simulink model "Stereotypes_Example"  (R2024a)
settings: Solver=VariableStepAuto  StartTime=0.0  StopTime=10.0  RelTol=1e-3
model workspace (MAT data in the model file):
  Var = 0
  architecture_gsCommands : Simulink.Bus (value not decoded)
  ctrlSrfcDeflection : Simulink.Bus (value not decoded)
  gs_commands_bus : Simulink.Bus (value not decoded)
  lightCmds : Simulink.Bus (value not decoded)
  mission_item_bus : Simulink.Bus (value not decoded)
  operatorCmds : Simulink.Bus (value not decoded)
  param_value_bus : Simulink.Bus (value not decoded)
(part 2 of 2)

== system Stereotypes_Example/Propulsion/Engine/ECU ==
  EFI : Subsystem
      settings: PortSchema="{\"entries\":[{\"content\":{\"headerSize\":26,\"margin\":15,\"minimumSpacing\":25,\"sides\":[{\"content\":{\"connectorIds\":[]},\"type\":\"ConnectorPlacement.EquallySpacedRectSide\",\"uuid\":\"288187f8-f80a-4535-8eff-6998f4e932c0\"},{\"content\":{\"connectorIds\":[\"Out1\"],\"side\":\"RIGHT\"},\"type\":\"ConnectorPlacement.EquallySpacedRectSide\",\"uuid\":\"d1e22774-cdd2-4e71-94b1-3e938d9d16f6\"},{\"content\":{\"connectorIds\":[],\"side\":\"TOP\"},\"type\":\"ConnectorPlacement.EquallySpacedRectSide\",\"uuid\":\"890411bd-a9cd-40b1-a683-0574f0cd14d7\"}]},\"type\":\"ConnectorPlacement.EquallySpacedConnector\",\"uuid\":\"f677e6f7-ddb0-43ad-ab3a-7892dac74d79\"}],\"packageUris\":[\"http:\\/\\/schema.mathworks.com\\/mf0\\/Connector\\/19700101\"],\"version\":\"1.0\"}"
  Bus Element Out1 : Outport  VectorParamsAs1DForOutWhenUnconnected=off  PortName=Engine Data

== system Stereotypes_Example/Propulsion/Engine/Engine ==
  Bus Element Out1 : Outport  VectorParamsAs1DForOutWhenUnconnected=off  PortName=Torque

== system Stereotypes_Example/Propulsion/Engine/Throttle Servo ==
  Bus Element In1 : Inport  PortName=dT

== system Stereotypes_Example/Propulsion/Fuel System/Fuel Filter ==
  Bus Element In1 : Inport  PortName=Fuel
  Bus Element Out1 : Outport  VectorParamsAs1DForOutWhenUnconnected=off  PortName=LP Fuel

== system Stereotypes_Example/Propulsion/Fuel System/Fuel Level Sensors ==
  Bus Element In1 : Inport  PortName=Fuel Level
  Bus Element Out1 : Outport  VectorParamsAs1DForOutWhenUnconnected=off  PortName=Signal

== system Stereotypes_Example/Propulsion/Fuel System/Fuel Pump ==
  Bus Element In1 : Inport  PortName=LP Fuel
  Bus Element Out1 : Outport  VectorParamsAs1DForOutWhenUnconnected=off  PortName=HP Fuel

== system Stereotypes_Example/Propulsion/Fuel System/Fuel Tank ==
  Bus Element In1 : Inport  PortName=Fuel Return LP
  Bus Element Out1 : Outport  VectorParamsAs1DForOutWhenUnconnected=off  PortName=Fuel
  Bus Element Out2 : Outport  Port=2  VectorParamsAs1DForOutWhenUnconnected=off  PortName=Fuel Level

== system Stereotypes_Example/Propulsion/Fuel System/Pressure Regulator ==
  Bus Element In1 : Inport  PortName=FuelReturn
  Bus Element Out1 : Outport  VectorParamsAs1DForOutWhenUnconnected=off  PortName=Fuel Return LP

== system Stereotypes_Example/Propulsion/Power Module/Backup Battery ==
  Bus Element Out1 : Outport  VectorParamsAs1DForOutWhenUnconnected=off  PortName=29V Battery

== system Stereotypes_Example/Propulsion/Power Module/Main Generator ==
  Bus Element In1 : Inport  PortName=MechConnection
  Bus Element Out1 : Outport  VectorParamsAs1DForOutWhenUnconnected=off  PortName=28V

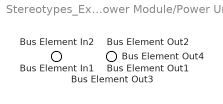
== system Stereotypes_Example/Propulsion/Power Module/Power Unit ==
  Bus Element In1 : Inport  PortName=28V
  Bus Element In2 : Inport  Port=2  PortName=29V Battery
  Bus Element Out1 : Outport  VectorParamsAs1DForOutWhenUnconnected=off  PortName=12V
  Bus Element Out2 : Outport  Port=2  VectorParamsAs1DForOutWhenUnconnected=off  PortName=24V
  Bus Element Out3 : Outport  Port=3  VectorParamsAs1DForOutWhenUnconnected=off  PortName=6V
  Bus Element Out4 : Outport  Port=4  VectorParamsAs1DForOutWhenUnconnected=off  PortName=Pwr Unit Status

== system Stereotypes_Example/Propulsion/Engine/ECU/EFI ==
  Bus Element Out1 : Outport  VectorParamsAs1DForOutWhenUnconnected=off  PortName=Engine Data
